simulink model "Math"  (R2015b)
settings: Solver=VariableStepAuto  StartTime=0.0  StopTime=20  RelTol=1e-3
settings Model: Creator=Druzhinin_Vasily  LastModifiedBy=User

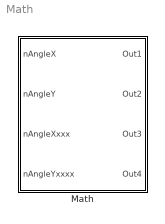
== system Math ==
  Math : Subsystem

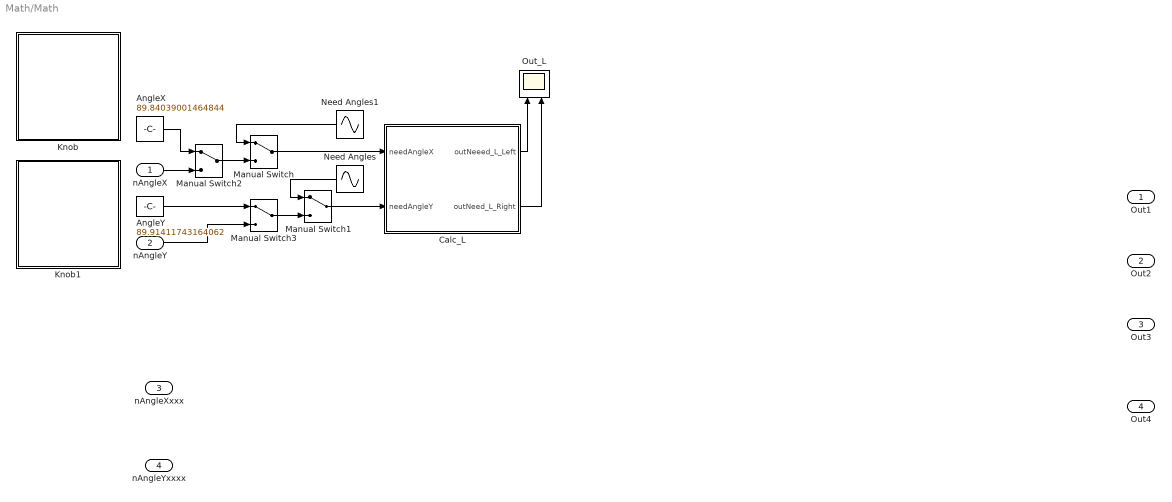
== system Math/Math ==
  nAngleX : Inport
  nAngleY : Inport  Port=2
  nAngleXxxx : Inport  Port=3
  nAngleYxxxx : Inport  Port=4
  AngleX : Constant  Value=89.84039001464844
  AngleY : Constant  Value=89.91411743164062
  Calc_L : MATLAB Function  TreatAsAtomicUnit=on
  Knob : Subsystem  DialogController=hmiCreateDDGDialog  IsWebBlock=on  mask(MWDashboardBlock){webBlockId=64e31e70-0dc6-4a47-9a86-7618526540fd, webBlockType=continuousknob, ShowInLibBrowser=on, ShowInitialText=on, HMISrcModelName=Math}
      mask prompts: webBlockId "WebBlock Id"; webBlockType "WebBlock Type"; HMISrcModelName "Source Model"
      mask Help: helpview([docroot '/mapfiles/simulink.map'], 'hmi_knob')
      mask Display:
      | if strcmp(get_param(bdroot(gcb),'BlockDiagramType'), 'library')
      |     image([(matlabroot) '/toolbox/simulink/hmi/icons/ContinuousKnob.png']);
      | end
  Knob1 : Subsystem  DialogController=hmiCreateDDGDialog  IsWebBlock=on  mask(MWDashboardBlock){webBlockId=c3abfad3-0788-43a3-9b1c-e570a5e0faec, webBlockType=continuousknob, ShowInLibBrowser=on, ShowInitialText=on, HMISrcModelName=Math}
      mask prompts: webBlockId "WebBlock Id"; webBlockType "WebBlock Type"; HMISrcModelName "Source Model"
      mask Help: helpview([docroot '/mapfiles/simulink.map'], 'hmi_knob')
      mask Display:
      | if strcmp(get_param(bdroot(gcb),'BlockDiagramType'), 'library')
      |     image([(matlabroot) '/toolbox/simulink/hmi/icons/ContinuousKnob.png']);
      | end
  Manual Switch{,1..3} (4 alike) : ManualSwitch
  Need Angles : Sin  Amplitude=20  Bias=90  SampleTime=0
  Need Angles1 : Sin  Amplitude=10  Bias=90  SampleTime=0
  Out_L : Scope  NumInputPorts=2
  Out1 : Outport
  Out2 : Outport  Port=2
  Out3 : Outport  Port=3
  Out4 : Outport  Port=4
  wires:
  Calc_L/1(outNeeed_L_Left) -> Out_L/1
  Calc_L/2(outNeed_L_Right) -> Out_L/2
  Need Angles/1 -> Manual Switch1/1
  Need Angles1/1 -> Manual Switch/1
  Manual Switch2/1 -> Manual Switch/2
  Manual Switch3/1 -> Manual Switch1/2
  Manual Switch1/1 -> Calc_L/2(needAngleY)
  Manual Switch/1 -> Calc_L/1(needAngleX)
  AngleX/1 -> Manual Switch2/1
  AngleY/1 -> Manual Switch3/1
  nAngleX/1 -> Manual Switch2/2
  nAngleY/1 -> Manual Switch3/2

== system Math/Math/Knob ==

== system Math/Math/Knob1 ==

== matlab function Math/Calc_L ==
  data: needAngleX input; outNeeed_L_Left output; needAngleY input; outNeed_L_Right output
function [outNeeed_L_Left,outNeed_L_Right] = fcn(needAngleX,needAngleY)
%#codegen

%Data
aX = 3;
bX = 4;

aY = 3;
bY = 4;

startL = 5;


%CalcL
L_fromOZD_Left_X  = Calc_L_UndoAlfa(aX,bX,needAngleX);
L_fromOZD_Right_X = Calc_L_UndoAlfa(aX,bX,needAngleX);

if (needAngleY<90)
    
    L_fromOZD_Left_Y  = startL - Calc_L_UndoAlfa(aY,bY,needAngleY);
    L_fromOZD_Right_Y = -1 *(startL - Calc_L_UndoAlfa(aY,bY,needAngleY));
    
elseif (needAngleY>90)
        
    L_fromOZD_Left_Y  = -1 * (startL - Calc_L_UndoAlfa(aY,bY,needAngleY));
    L_fromOZD_Right_Y = startL - Calc_L_UndoAlfa(aY,bY,needAngleY);
    
else
    L_fromOZD_Left_Y  = 0;
    L_fromOZD_Right_Y = 0;
end;
    

outNeeed_L_Left = L_fromOZD_Left_X + L_fromOZD_Left_Y;
outNeed_L_Right = L_fromOZD_Right_X + L_fromOZD_Right_Y;
